simulink model "cantoni_combined_matrices_ETC"  (R2019a)
settings: Solver=VariableStepAuto  StartTime=0.0  StopTime=2000  FixedStep=h  RelTol=1e-3
InitFcn:
  | ini_cantonisim_distributed
values from neighbouring files (symbols this model uses):
  comb_contr = ss(Ac, Bc, Cc, Dc, h)    [cantoni_LMI.m]
  comb_plant_cont = ss(Ap, Bp, Cp, Dp)    [cantoni_LMI.m]
  h = 1    [cantoni_LMI.m]    (also in distributed_workspace.mat; model_hil.m = 0.00208333333333)
undefined symbols (not defined in the file or in its folder): DiscIntNeverNeededParam, sigma
settings Model: Creator=Jacob  LastModifiedBy=Jacob

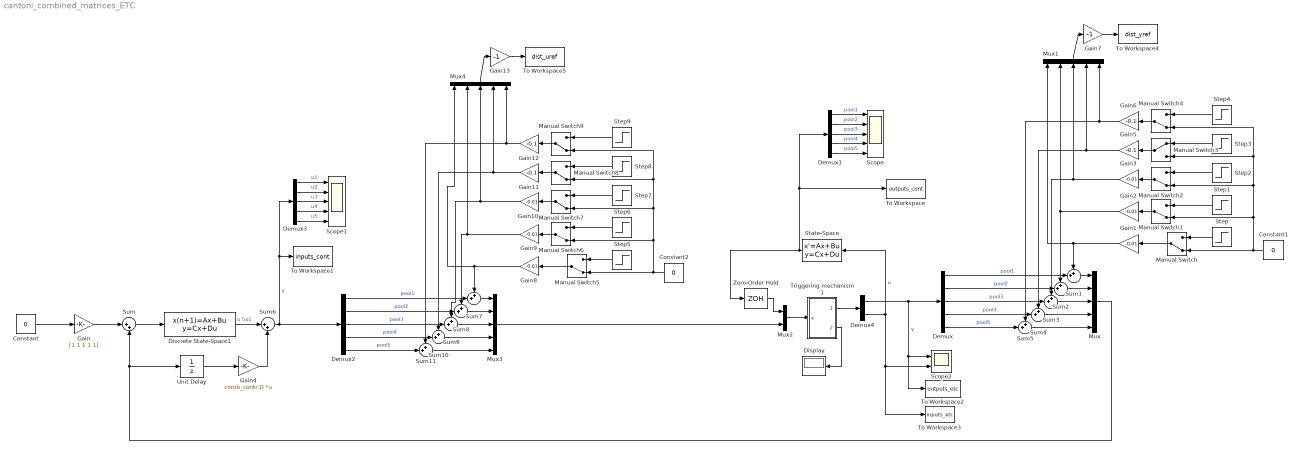
== system cantoni_combined_matrices_ETC ==
  Constant : Constant  Value=0
  Constant1 : Constant  Value=0
  Constant2 : Constant  Value=0
  Demux{,1..3} (4 alike) : Demux  Outputs=5
  Demux4 : Demux  Outputs=2
  Discrete State-Space1 : DiscreteStateSpace  A=comb_contr.A  B=comb_contr.B  C=comb_contr.C  D=comb_contr.D*0  SampleTime=h
  Display : Display
  Gain : Gain  Gain=[1 1 1 1 1]
  Gain{1..3,8..10} (6 alike) : Gain  Gain=-0.01
  Gain{5..6,11..12} (4 alike) : Gain  Gain=-0.1
  Gain13 : Gain  Gain=-1
  Gain4 : Gain  Gain=comb_contr.D  Multiplication=Matrix(K*u)
  Gain7 : Gain  Gain=-1
  Manual Switch{,1..2,4..9} (9 alike) : ManualSwitch  CurrentSetting=0
  Manual Switch3 : ManualSwitch
  Mux{,1,3..4} (4 alike) : Mux  Inputs=5
  Mux2 : Mux  Inputs=2
  Scope : Scope  NumInputPorts=5
  Scope1 : Scope  NumInputPorts=5
  Scope2 : Scope  NumInputPorts=2
  State-Space : StateSpace  A=comb_plant_cont.A  B=comb_plant_cont.B  C=comb_plant_cont.C  D=comb_plant_cont.D  InitialCondition=0
  Step{,1..9} (10 alike) : Step  Time=50  SampleTime=0
  Sum : Sum  Inputs=|++
  Sum{1..5,7..11} (10 alike) : Sum  Inputs=++|
  Sum6 : Sum  Inputs=|++
  To Workspace : ToWorkspace  VariableName=outputs_cont  SaveFormat=Timeseries  SampleTime=-1
  To Workspace1 : ToWorkspace  VariableName=inputs_cont  SaveFormat=Timeseries  SampleTime=-1
  To Workspace2 : ToWorkspace  VariableName=outputs_etc  SaveFormat=Timeseries  SampleTime=-1
  To Workspace3 : ToWorkspace  VariableName=inputs_etc  SaveFormat=Timeseries  SampleTime=-1
  To Workspace4 : ToWorkspace  VariableName=dist_yref  SaveFormat=Timeseries  SampleTime=-1
  To Workspace5 : ToWorkspace  VariableName=dist_uref  SaveFormat=Timeseries  SampleTime=-1
  Triggering mechanism 1 : Subsystem
  Unit Delay : UnitDelay  SampleTime=-1  HasFrameUpgradeWarning=on
  Zero-Order Hold : ZeroOrderHold  SampleTime=h
  wires:
  Sum/1 -> Discrete State-Space1/1
  Constant/1 -> Gain/1
  Gain/1 -> Sum/1
  Demux1/1 -> Scope/1  "pool1"
  Demux1/2 -> Scope/2  "pool2"
  Demux1/3 -> Scope/3  "pool3"
  Demux1/4 -> Scope/4  "pool4"
  Demux1/5 -> Scope/5  "pool5"
  Step/1 -> Manual Switch/1
  Sum1/1 -> Mux/1
  Demux/2 -> Sum2/2  "pool2"
  Sum2/1 -> Mux/2
  Gain2/1 -> Mux1/2, Sum2/1
  Step1/1 -> Manual Switch1/1
  Gain1/1 -> Mux1/1, Sum1/1
  Manual Switch/1 -> Gain1/1
  Constant1/1 -> Manual Switch1/2, Manual Switch4/2, Manual Switch3/2, Manual Switch2/2, Manual Switch/2
  Manual Switch1/1 -> Gain2/1
  Demux/3 -> Sum3/2  "pool3"
  Sum3/1 -> Mux/3
  Manual Switch2/1 -> Gain3/1
  Step2/1 -> Manual Switch2/1
  Gain3/1 -> Sum3/1, Mux1/3
  Demux/1 -> Sum1/2  "pool1"
  Demux/4 -> Sum4/2  "pool4"
  Sum4/1 -> Mux/4
  Demux/5 -> Sum5/2  "pool5"
  Sum5/1 -> Mux/5
  Step3/1 -> Manual Switch3/1
  Manual Switch3/1 -> Gain5/1
  Gain5/1 -> Mux1/4, Sum4/1
  Manual Switch4/1 -> Gain6/1
  Step4/1 -> Manual Switch4/1
  Gain6/1 -> Mux1/5, Sum5/1
  Discrete State-Space1/1 -> Sum6/1  "u 5x1"
  Demux3/5 -> Scope1/5  "u5"
  Demux3/4 -> Scope1/4  "u4"
  Demux3/3 -> Scope1/3  "u3"
  Demux3/2 -> Scope1/2  "u2"
  Demux3/1 -> Scope1/1  "u1"
  Triggering mechanism 1/1(xhat) -> Demux4/1
  Mux2/1 -> Triggering mechanism 1/1(x)
  Mux/1 -> Sum/2, Unit Delay/1
  Triggering mechanism 1/2(Comm count) -> Display/1
  Zero-Order Hold/1 -> Mux2/1
  State-Space/1 -> Zero-Order Hold/1, Demux1/1, To Workspace/1
  Demux4/1 -> To Workspace2/1, Scope2/1, Demux/1  "y"
  Demux4/2 -> State-Space/1, To Workspace3/1, Scope2/2  "u"
  Unit Delay/1 -> Gain4/1
  Gain4/1 -> Sum6/2
  Gain7/1 -> To Workspace4/1
  Mux1/1 -> Gain7/1
  Demux2/4 -> Sum10/2  "pool4"
  Sum6/1 -> Demux2/1, To Workspace1/1, Demux3/1  "y"
  Sum10/1 -> Mux3/4
  Demux2/5 -> Sum11/2  "pool5"
  Demux2/2 -> Sum8/2  "pool2"
  Sum11/1 -> Mux3/5
  Sum9/1 -> Mux3/3
  Demux2/1 -> Sum7/2  "pool1"
  Demux2/3 -> Sum9/2  "pool3"
  Sum7/1 -> Mux3/1
  Sum8/1 -> Mux3/2
  Mux3/1 -> Mux2/2
  Manual Switch7/1 -> Gain10/1
  Manual Switch8/1 -> Gain11/1
  Step7/1 -> Manual Switch7/1
  Step8/1 -> Manual Switch8/1
  Step5/1 -> Manual Switch5/1
  Gain12/1 -> Sum11/1, Mux4/5
  Step9/1 -> Manual Switch9/1
  Manual Switch9/1 -> Gain12/1
  Gain10/1 -> Sum9/1, Mux4/3
  Gain11/1 -> Sum10/1, Mux4/4
  Constant2/1 -> Manual Switch6/2, Manual Switch9/2, Manual Switch8/2, Manual Switch7/2, Manual Switch5/2
  Gain9/1 -> Sum8/1, Mux4/2
  Step6/1 -> Manual Switch6/1
  Gain8/1 -> Sum7/1, Mux4/1
  Mux4/1 -> Gain13/1
  Gain13/1 -> To Workspace5/1
  Manual Switch6/1 -> Gain9/1
  Manual Switch5/1 -> Gain8/1

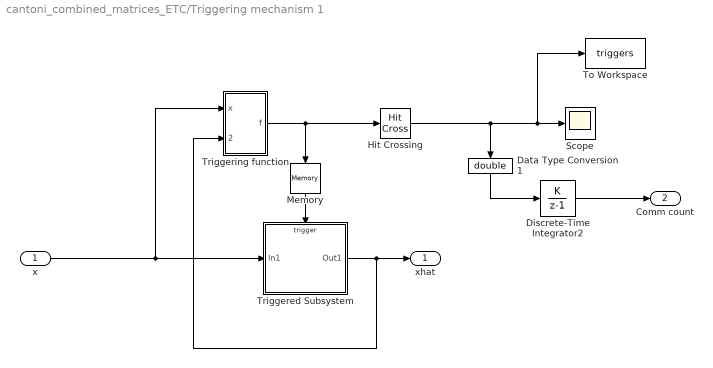
== system cantoni_combined_matrices_ETC/Triggering mechanism 1 ==
  x : Inport
  Data Type Conversion1 : DataTypeConversion  OutDataTypeStr=double
  Discrete-Time Integrator2 : DiscreteIntegrator  IntegratorMethod=Accumulation: Forward Euler  gainval=1  SampleTime=-1  ICPrevOutput=DiscIntNeverNeededParam  ICPrevScaledInput=DiscIntNeverNeededParam
  Hit Crossing : HitCross  HitCrossingDirection=rising
  Memory : Memory
  Scope : Scope
  To Workspace : ToWorkspace  VariableName=triggers  SaveFormat=Timeseries  SampleTime=-1
  Triggered Subsystem : Subsystem  TreatAsAtomicUnit=on
  Triggering function : Subsystem
  xhat : Outport
  Comm count : Outport  Port=2
  wires:
  Hit Crossing/1 -> Data Type Conversion1/1, To Workspace/1, Scope/1
  Triggered Subsystem/1(Out1) -> Triggering function/2(xhat), xhat/1
  Triggering function/1(f) -> Memory/1, Hit Crossing/1
  Memory/1 -> Triggered Subsystem/Trigger
  x/1 -> Triggered Subsystem/1(In1), Triggering function/1(x)
  Data Type Conversion1/1 -> Discrete-Time Integrator2/1
  Discrete-Time Integrator2/1 -> Comm count/1

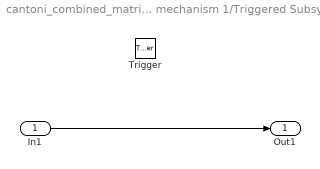
== system cantoni_combined_matrices_ETC/Triggering mechanism 1/Triggered Subsystem ==
  In1 : Inport
  Trigger : TriggerPort  VariantControl=Variant  InitialTriggerSignalState=negative
  Out1 : Outport
  wires:
  In1/1 -> Out1/1

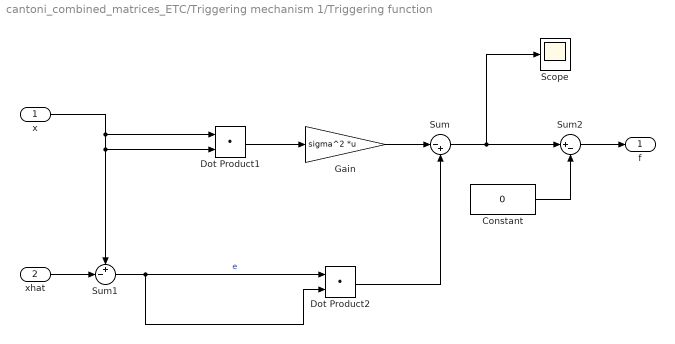
== system cantoni_combined_matrices_ETC/Triggering mechanism 1/Triggering function ==
  x : Inport
  xhat : Inport  Port=2
  Constant : Constant  Value=0
  Dot Product1 : DotProduct  InputSameDT=on  OutDataTypeStr=Inherit: Inherit via internal rule
  Dot Product2 : DotProduct  InputSameDT=on  OutDataTypeStr=Inherit: Inherit via internal rule
  Gain : Gain  Gain=sigma^2  Multiplication=Matrix(K*u)
  Scope : Scope
  Sum : Sum  Inputs=|-+
  Sum1 : Sum  Inputs=+-|
  Sum2 : Sum  Inputs=|+-
  f : Outport
  wires:
  xhat/1 -> Sum1/2
  Gain/1 -> Sum/1
  Sum1/1 -> Dot Product2/2, Dot Product2/1  "e"
  Dot Product2/1 -> Sum/2
  Sum/1 -> Sum2/1, Scope/1
  x/1 -> Dot Product1/1, Dot Product1/2, Sum1/1
  Sum2/1 -> f/1
  Constant/1 -> Sum2/2
  Dot Product1/1 -> Gain/1
